simulink model "carmen_controller_forced"  (Simulink 8.2)
settings: Solver=FixedStepDiscrete  SolverMode=SingleTasking  StartTime=0.0  StopTime=inf  RelTol=1e-3
PreLoadFcn:
  | waijung.modelPreload; % Required for working with Waijung Blockset. Do not remove.
undefined symbols (not defined in the file or in its folder): ARM, Link, LQFP100, MDK, ST, STM32F407VG, STM32F4DISCOVERY
libraries: simulink x4, BC_USB x2, stm32f4_adc_lib x1, stm32f4_io_lib x1, stm32f4_device_config_lib x1
CloseFcn:
  | waijung.modelClose; % Required for working with Waijung Blockset. Do not remove.
settings Model: Creator=Sr Antonio  LastModifiedBy=Cristina
settings OptimizationCC: OptimizeModelRefInitCode=on  LifeSpan=1
settings DebuggingCC: FcnCallInpInsideContextMsg=EnableAllAsWarning
settings HardwareCC: ProdEndianess=LittleEndian  ProdHWDeviceType=ARM Compatible->Cortex - M4  TargetEndianess=LittleEndian  TargetHWDeviceType=ARM Compatible->Cortex - M4
settings RTWCC: SystemTargetFile=stm32f4.tlc  GenerateMakefile=off  TemplateMakefile=ert_default_tmf  Description=STM32F4 Target  ProcessScript=stm32f4_make_rtw_hook
settings CodeAppCC: IgnoreCustomStorageClasses=off  CustomSymbolStrType=$N$R$M  InternalIdentifier=Classic
settings STFCustomTargetCC: CodeReplacementLibrary=ANSI_C  ModelReferenceCompliant=off  CombineOutputUpdateFcns=on  ERTCustomFileBanners=on  SupportContinuousTime=off  SupportNonInlinedSFcns=off  MATLABClassNameForMDSCustomization=Simulink.SoftwareTarget.ERTCustomization  GRTInterface=off  SystemTargetFile=stm32f4.tlc
settings ERTTargetCC: CodeReplacementLibrary=ANSI_C  MultiwordLength=2048  ModelReferenceCompliant=off  ParMdlRefBuildCompliant=off  CompOptLevelCompliant=off  ConcurrentExecutionCompliant=off  ERTFirstTimeCompliant=off  ModelStepFunctionPrototypeControlCompliant=off  CPPClassGenCompliant=off  ExtModeMexFile=noextcomm  InlinedParameterPlacement=NonHierarchical  ERTSrcFileBannerTemplate=stm32f4_code_template.cgt  ERTHdrFileBannerTemplate=stm32f4_code_template.cgt  ERTDataSrcFileTemplate=stm32f4_code_template.cgt  ERTDataHdrFileTemplate=stm32f4_code_template.cgt  ERTCustomFileTemplate=stm32f4_file_process.tlc  ConvertIfToSwitch=off  SuppressUnreachableDefaultCases=off

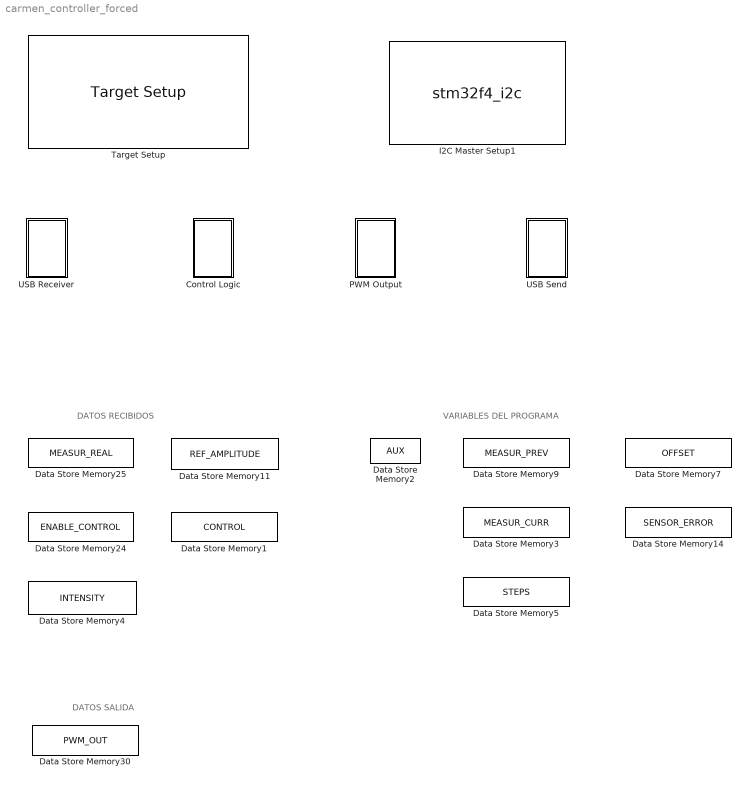
== system carmen_controller_forced ==
  note: VARIABLES DEL PROGRAMA
  note: DATOS RECIBIDOS
  note: DATOS SALIDA
  Control Logic : Subsystem  Priority=2
  Data Store Memory1 : DataStoreMemory  DataStoreName=CONTROL  ReadBeforeWriteMsg=warning  WriteAfterWriteMsg=warning  WriteAfterReadMsg=warning  OutDataTypeStr=single
  Data Store Memory11 : DataStoreMemory  DataStoreName=REF_AMPLITUDE  ReadBeforeWriteMsg=warning  WriteAfterWriteMsg=warning  WriteAfterReadMsg=warning  InitialValue=single(0)  OutDataTypeStr=single
  Data Store Memory14 : DataStoreMemory  DataStoreName=SENSOR_ERROR  ReadBeforeWriteMsg=warning  WriteAfterWriteMsg=warning  WriteAfterReadMsg=warning  OutDataTypeStr=uint8
  Data Store Memory2 : DataStoreMemory  DataStoreName=AUX  ReadBeforeWriteMsg=warning  WriteAfterWriteMsg=warning  WriteAfterReadMsg=warning  OutDataTypeStr=uint8
  Data Store Memory24 : DataStoreMemory  DataStoreName=ENABLE_CONTROL  ReadBeforeWriteMsg=warning  WriteAfterWriteMsg=warning  WriteAfterReadMsg=warning  OutDataTypeStr=uint8
  Data Store Memory25 : DataStoreMemory  DataStoreName=MEASUR_REAL  ReadBeforeWriteMsg=warning  WriteAfterWriteMsg=warning  WriteAfterReadMsg=warning  OutDataTypeStr=int32
  Data Store Memory3 : DataStoreMemory  DataStoreName=MEASUR_CURR  ReadBeforeWriteMsg=warning  WriteAfterWriteMsg=warning  WriteAfterReadMsg=warning  OutMin=0  OutMax=4096  OutDataTypeStr=uint16
  Data Store Memory30 : DataStoreMemory  DataStoreName=PWM_OUT  ReadBeforeWriteMsg=warning  WriteAfterWriteMsg=warning  WriteAfterReadMsg=warning  OutDataTypeStr=single
  Data Store Memory4 : DataStoreMemory  DataStoreName=INTENSITY  ReadBeforeWriteMsg=warning  WriteAfterWriteMsg=warning  WriteAfterReadMsg=warning  OutDataTypeStr=single
  Data Store Memory5 : DataStoreMemory  DataStoreName=STEPS  ReadBeforeWriteMsg=warning  WriteAfterWriteMsg=warning  WriteAfterReadMsg=warning  OutDataTypeStr=int8
  Data Store Memory7 : DataStoreMemory  DataStoreName=OFFSET  ReadBeforeWriteMsg=warning  WriteAfterWriteMsg=warning  WriteAfterReadMsg=warning  InitialValue=150  OutDataTypeStr=uint16
  Data Store Memory9 : DataStoreMemory  DataStoreName=MEASUR_PREV  ReadBeforeWriteMsg=warning  WriteAfterWriteMsg=warning  WriteAfterReadMsg=warning  OutMin=0  OutMax=4096  OutDataTypeStr=uint16
  I2C Master Setup1 : S-Function  Priority=2  FunctionName=stm32f4_i2c  Parameters=configuration,module,transfer,clkspeed,timeout,sdapin,sclpin,writecount,readcount,inputtypearray,outputtypearray,confstr,sampletime,sampletimestr,blockid  EnableBusSupport=off  mask(stm32f4_i2c){configuration=Setup, module=1, lastmodule=1, transfer=Blocking, dutycycle=TLow/THigh = 2, clkspeed=600, timeout=1, writecount=0, readcount=0, sdapin=B9, sclpin=B8, waitwritetime=0, inputtypearray=[0], outputtypearray=[0], confstr=["B","9","B","8","1","1","6","0","I2C_DutyCycle_2","0","off"], sampletime=-1, sampletimestr=0.002, blockid=I2CMasterSetup1}
      mask prompts: module "I2C Module"; lastmodule "Last module"; transfer "Transfer mode"; dutycycle "Duty cycle in fast mode"; clkspeed "Clock speed (kHz)"; timeout "Timeout (ms)"; writecount "Bytes write count"; readcount "Bytes read count"; sdapin "SDA pin"; sclpin "SCL pin"; waitwritetime "Wait write time (ms), default is 0"; inputtypearray "Input type array"; outputtypearray "Output type array"; confstr "Configuration string"; sampletime "Sample time (sec)"; sampletimestr "Compiled sample time (sec) in string"
      mask init:
      | stm32f4_i2c_callback('init');
      mask Help: web(fullfile(waijungdocroot,'stm32f4_i2c_setup.htm'), '-browser')
      mask TypeOptions configuration: Setup | Transaction
      mask Callback configuration: stm32f4_i2c_callback('configuration');
      mask TypeOptions module: 1 | 2 | 3
      mask Callback module: stm32f4_i2c_callback('module');
      mask TypeOptions transfer: Blocking | Non-blocking
      mask TypeOptions dutycycle: TLow/THigh = 16/9 | TLow/THigh = 2
      mask Callback dutycycle: stm32f4_i2c_callback('dutycycle');
      mask Callback writecount: stm32f4_i2c_callback('writecount');
      mask Callback readcount: stm32f4_i2c_callback('readcount');
      mask TypeOptions sdapin: - | B7 | B9
      mask Callback sdapin: stm32f4_i2c_callback('sdapin');
      mask TypeOptions sclpin: - | B6 | B8
      mask Callback sclpin: stm32f4_i2c_callback('sclpin');
      mask Callback confstr: stm32f4_i2c_callback('confstr');
      mask Callback sampletime: stm32f4_i2c_callback('sampletime');
      mask Callback sampletimestr: stm32f4_i2c_callback('sampletimestr');
      mask Callback blockid: stm32f4_i2c_callback('blockid');
      mask Display: text(0.5, 0.5, 'Module: I2C1\nClock: 600kHz\nSDA/SCL Pin: B9/B8','ver','middle','hor','center');
  PWM Output : Subsystem  Priority=3
  Target Setup : stm32f4_device_config_lib/Target Setup  Priority=1  compiler=MDK-ARM  previous_compiler=MDK-ARM  mcu=STM32F407VG (LQFP100); STM32F4DISCOVERY  mcustr=STM32F407VG  clockconfig=STM32F4DISCOVERY Default (HSEOSC-8MHz/HCLK-168MHz)  system_stm32f4xx_c_path=C:\BC_3\targets\stm32f4_target\stm32f4\utils\STM32F4xx_AN3988_V1.0.1\stm32f4_default\hseosc8mhz  showmemoryconfiguration=on  stacksize=0x1600  heapsize=0x1600  enableautocompiledownload=on  fullchiperase=off  programmerinterface=ST-Link  editctrlstr=on  compilercontrolstr=-c --cpu Cortex-M4.fp -g -O3 --apcs=interwork --split_sections $(INCLUDES)  assemblercontrolstr="--cpu Cortex-M4.fp -g --apcs=interwork  --xref $(INCLUDES)"  linkercontrolstr="--cpu Cortex-M4.fp --strict --scatter \"$(MODELNAME).sct\" --summary_stderr --info summarysizes --map --xref --callgraph --symbols --info sizes --info totals --info unused --info veneers  --list \".\\$(MODELNAME).map\" -o $(MODELNAME).axf"  runafterdownload=on  execprofile=None  profileruart=3  profilerbaud=500000  profilertxpin=D8  profilerinitstr=0.002,168000000,336000,500000,0  manualsetsampletime=on  sampletime=0.002  blockid=TargetSetup  systickreloadvalue=336000  hseval=8000000  lastprofileruart=3  hclk=168000000  flashorigin=0x08000000  flashlength=0x00100000  ramorigin=0x20000000  ramlength=0x00020000  useextram=off
  USB Receiver : Subsystem  Priority=4
  USB Send : Subsystem  Priority=5

== system carmen_controller_forced/Control Logic ==
  Read Sensor : Subsystem  Priority=2

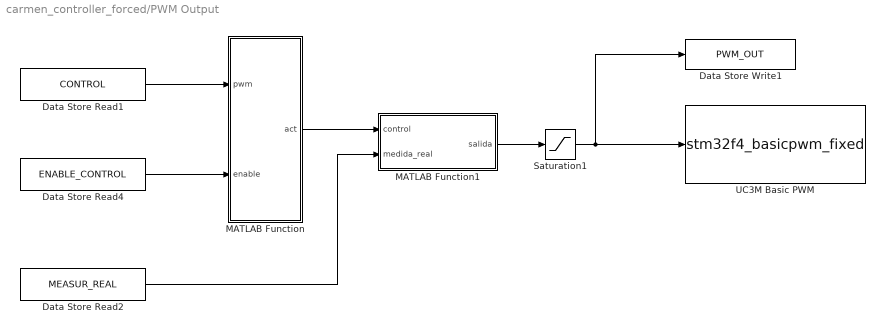
== system carmen_controller_forced/PWM Output ==
  Data Store Read1 : DataStoreRead  DataStoreName=CONTROL
  Data Store Read2 : DataStoreRead  DataStoreName=MEASUR_REAL
  Data Store Read4 : DataStoreRead  DataStoreName=ENABLE_CONTROL
  Data Store Write1 : DataStoreWrite  DataStoreName=PWM_OUT
  MATLAB Function : MATLAB Function  TreatAsAtomicUnit=on
  MATLAB Function1 : MATLAB Function  TreatAsAtomicUnit=on
  Saturation1 : Saturate  UpperLimit=100  LowerLimit=0  OutDataTypeStr=single
  UC3M Basic PWM : S-Function  Priority=6  FunctionName=stm32f4_basicpwm_fixed  Parameters=timer,pwmperiod,uc3m_pwmperiod,ch1pin,ch2pin,ch3pin,ch4pin,sampletime,sampletimestr,blockid,apb,portstr,pinstr,pinmat,timarr,timprescale,chmat,polaritystr  EnableBusSupport=off  mask(stm32f4_basicpwm_fixed){timer=2, pwmperiod=0.02, uc3m_pwmperiod=0.001, polarity=Active High, polaritystr=TIM_OCPolarity_High, ch1pin=Not available - Do not use, ch2pin=B3, ch3pin=Not available - Do not use, ch4pin=Not available - Do not use, sampletime=0.002, sampletimestr=0, blockid=PWMOutputUC3MBasicPWM, portpinstr=,B3,,, enablecustomportlabel=off, cinputportlabel=In1, In2, In3, In4, coutputportlabel=0, callbackgensrccode=off, apb=1, portstr=["B"], pinstr=["GPIO_Pin_3"], pinmat=[1 3], timarr=59999, timprescale=55, chmat=[2]}
      mask prompts: pwmperiod "PWM Period (seconds)"; uc3m_pwmperiod "PWM Signal Period (seconds)"; ch1pin "Channel 1"; ch2pin "Channel 2"; ch3pin "Channel 3"; ch4pin "Channel 4"; sampletime "Sample time (sec)"; sampletimestr "Compiled sample time (sec) in string"; portpinstr "Port pin string"; enablecustomportlabel "Enable custom port labels"; cinputportlabel "Custom input port labels (Ex. In1, In2, In3)"; coutputportlabel "Custom output port labels (Ex. Out1, Out2, Out3)"; callbackgensrccode "Gen source code from callback"; portstr "Port string"; pinstr "Pin string"; pinmat "Pin matrix"; timarr "Timer ARR"; timprescale "Timer PRESCALE"; chmat "Channel order"
      mask help:
      | This block implements basic Edge-aligned Pulse Width Modulation (PWM) generation.
      | All timers are 16-bit. The PWM period is fixed (per timer).
      |
      | This block was fixed by Sr Antonio
      mask init:
      | stm32f4_basicpwm_callback_fixed('init');
      mask Help: web(fullfile(waijungdocroot,'stm32f4_basicpwm.htm'),'-browser')
      mask TypeOptions timer: 1 | 2 | 3 | 4 | 5 | 8 | 9 | 10 | 11 | 12 | 13 | 14
      mask Callback timer: stm32f4_basicpwm_callback_fixed('timer');
      mask Callback pwmperiod: stm32f4_basicpwm_callback_fixed('pwmperiod');
      mask Callback uc3m_pwmperiod: stm32f4_basicpwm_callback_fixed('uc3m_pwmperiod');
      mask TypeOptions polarity: Active High | Active Low
      mask Callback polarity: stm32f4_basicpwm_callback_fixed('polarity');
      mask TypeOptions ch1pin: Not available - Do not use | A0 | A5
      mask Callback ch1pin: stm32f4_basicpwm_callback_fixed('ch1pin');
      mask TypeOptions ch2pin: Not available - Do not use | A1 | B3
      mask Callback ch2pin: stm32f4_basicpwm_callback_fixed('ch2pin');
      mask TypeOptions ch3pin: Not available - Do not use | A2 | B10
      mask Callback ch3pin: stm32f4_basicpwm_callback_fixed('ch3pin');
      mask TypeOptions ch4pin: Not available - Do not use | A3 | B11
      mask Callback ch4pin: stm32f4_basicpwm_callback_fixed('ch4pin');
      mask Callback sampletime: stm32f4_basicpwm_callback_fixed('sampletime');
      mask Callback sampletimestr: stm32f4_basicpwm_callback_fixed('sampletimestr');
      mask Callback blockid: stm32f4_basicpwm_callback_fixed('blockid');
      mask Callback enablecustomportlabel: stm32f4_basicpwm_callback_fixed('enablecustomportlabel')
      mask Display: text(0.95, 0.5, 'UC3M FIXED\nTimer: 2\nPolarity: Active High\nPeriod (sec): 0.001\nTs (sec): 0.002','ver','middle','hor','right');port_label('input', 1,'CH2 (B3)')
  wires:
  Data Store Read1/1 -> MATLAB Function/1(pwm)
  Data Store Read4/1 -> MATLAB Function/2(enable)
  MATLAB Function/1(act) -> MATLAB Function1/1(control)
  Saturation1/1 -> UC3M Basic PWM/1, Data Store Write1/1
  Data Store Read2/1 -> MATLAB Function1/2(medida_real)
  MATLAB Function1/1(salida) -> Saturation1/1

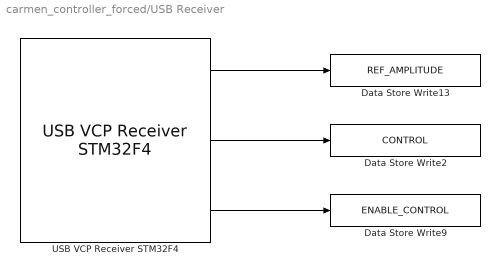
== system carmen_controller_forced/USB Receiver ==
  Data Store Write13 : DataStoreWrite  DataStoreName=REF_AMPLITUDE
  Data Store Write2 : DataStoreWrite  DataStoreName=CONTROL
  Data Store Write9 : DataStoreWrite  DataStoreName=ENABLE_CONTROL
  USB VCP Receiver STM32F4 : BC_USB/USB VCP Receiver STM32F4  speed="USB 1.1   12Mbit/s"  data_size=2048 Bytes  header_data='0E 0E'  binary_data='single single uint8'  terminator_data='0A 0A'  sampletime=0.01
  wires:
  USB VCP Receiver STM32F4/1 -> Data Store Write13/1
  USB VCP Receiver STM32F4/2 -> Data Store Write2/1
  USB VCP Receiver STM32F4/3 -> Data Store Write9/1

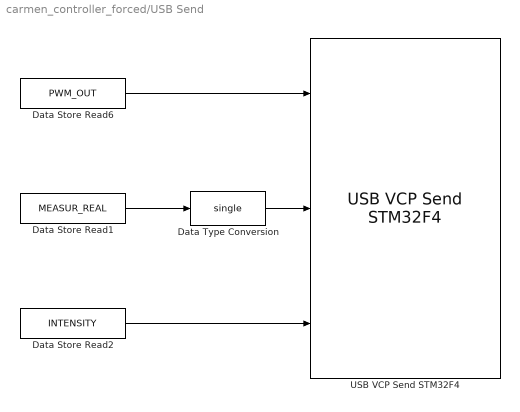
== system carmen_controller_forced/USB Send ==
  Data Store Read1 : DataStoreRead  DataStoreName=MEASUR_REAL  SampleTime=0.002
  Data Store Read2 : DataStoreRead  DataStoreName=INTENSITY  SampleTime=0.01
  Data Store Read6 : DataStoreRead  DataStoreName=PWM_OUT  SampleTime=0.002
  Data Type Conversion : DataTypeConversion  OutDataTypeStr=single
  USB VCP Send STM32F4 : BC_USB/USB VCP Send STM32F4  speed="USB 1.1   12Mbit/s"  data_size=2048 Bytes  header_data='0E 0E'  binary_data='single single single'  terminator_data='0A 0A'  sampletime=0.01
  wires:
  Data Store Read1/1 -> Data Type Conversion/1
  Data Store Read6/1 -> USB VCP Send STM32F4/1
  Data Type Conversion/1 -> USB VCP Send STM32F4/2
  Data Store Read2/1 -> USB VCP Send STM32F4/3

== system carmen_controller_forced/Control Logic/Read Sensor ==
  note: LECTURA DEL SENSOR DE INTENSIDAD
  note: CÁLCULO DE LA POSICIÓN REAL DEL ACTUADOR
  note: LECTURA DEL SENSOR DE POSICIÓN
  Calculate the SMA real position : Subsystem  Priority=3
  Intensity Readout : Subsystem  Priority=2
  Sensor Readout : Subsystem  Priority=2

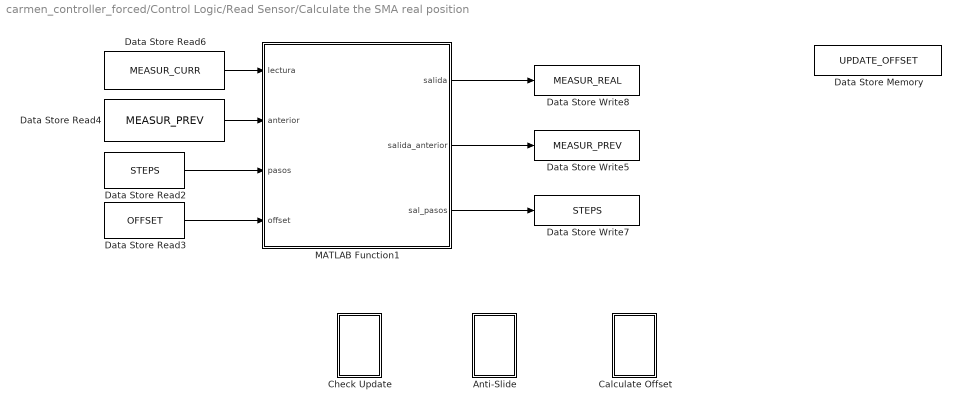
== system carmen_controller_forced/Control Logic/Read Sensor/Calculate the SMA real position ==
  Anti-Slide : Subsystem  Priority=51
  Calculate Offset : Subsystem  Priority=52
  Check Update : Subsystem  Priority=50
  Data Store Memory : DataStoreMemory  DataStoreName=UPDATE_OFFSET  ReadBeforeWriteMsg=warning  WriteAfterWriteMsg=warning  WriteAfterReadMsg=warning  OutDataTypeStr=uint8
  Data Store Read2 : DataStoreRead  DataStoreName=STEPS  SampleTime=0.002
  Data Store Read3 : DataStoreRead  DataStoreName=OFFSET  SampleTime=0.002
  Data Store Read4 : DataStoreRead  DataStoreName=MEASUR_PREV  SampleTime=0.002
  Data Store Read6 : DataStoreRead  DataStoreName=MEASUR_CURR  SampleTime=0.002
  Data Store Write5 : DataStoreWrite  DataStoreName=MEASUR_PREV  SampleTime=0.002
  Data Store Write7 : DataStoreWrite  DataStoreName=STEPS  SampleTime=0.002
  Data Store Write8 : DataStoreWrite  DataStoreName=MEASUR_REAL  SampleTime=0.002
  MATLAB Function1 : MATLAB Function  TreatAsAtomicUnit=on
  wires:
  Data Store Read2/1 -> MATLAB Function1/3(pasos)
  Data Store Read4/1 -> MATLAB Function1/2(anterior)
  MATLAB Function1/3(sal_pasos) -> Data Store Write7/1
  Data Store Read6/1 -> MATLAB Function1/1(lectura)
  MATLAB Function1/1(salida) -> Data Store Write8/1
  MATLAB Function1/2(salida_anterior) -> Data Store Write5/1
  Data Store Read3/1 -> MATLAB Function1/4(offset)

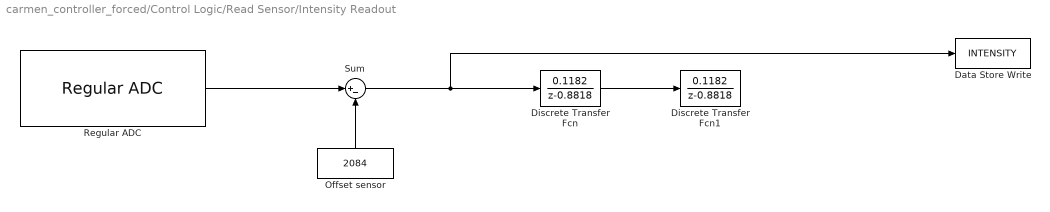
== system carmen_controller_forced/Control Logic/Read Sensor/Intensity Readout ==
  Data Store Write : DataStoreWrite  DataStoreName=INTENSITY
  Discrete Transfer Fcn : DiscreteTransferFcn  Numerator=[0.1182]  Denominator=[1 -0.8818]
  Discrete Transfer Fcn1 : DiscreteTransferFcn  Numerator=[0.1182]  Denominator=[1 -0.8818]
  Offset sensor : Constant  Value=2084  OutDataTypeStr=single
  Regular ADC : stm32f4_adc_lib/Regular ADC  adcmodule=1  outputdatatype=Single  prescaler=2  prescalerstr=ADC_Prescaler_Div2  chsamplingtime=Auto  chsamplingtimestr=ADC_SampleTime_480Cycles  read_an0=off  read_an1=off  read_an2=on  read_an3=off  read_an4=off  read_an5=off  read_an6=off  read_an7=off  read_an8=off  read_an9=off  read_an10=off  read_an11=off  read_an12=off  read_an13=off  read_an14=off  read_an15=off  read_an16=off  read_an17=off  read_an18=off  pinstr=GPIO_Pin_2  usedpinarray="[0  0  1  0  0  0  0  0  0  0  0  0  0  0  0  0  0  0  0]"  usedportidarray=[0]  usedpinidarray=[2]  usedpinidcount=1  sampletime=0.002  blockid=ControlLogicReadSensorIntensityReadoutRegularADC  enablecustomportlabel=off  cinputportlabel=0  coutputportlabel=Out1, Out2
  Sum : Sum  Inputs=|+-
  wires:
  Discrete Transfer Fcn/1 -> Discrete Transfer Fcn1/1
  Regular ADC/1 -> Sum/1
  Sum/1 -> Data Store Write/1, Discrete Transfer Fcn/1
  Offset sensor/1 -> Sum/2

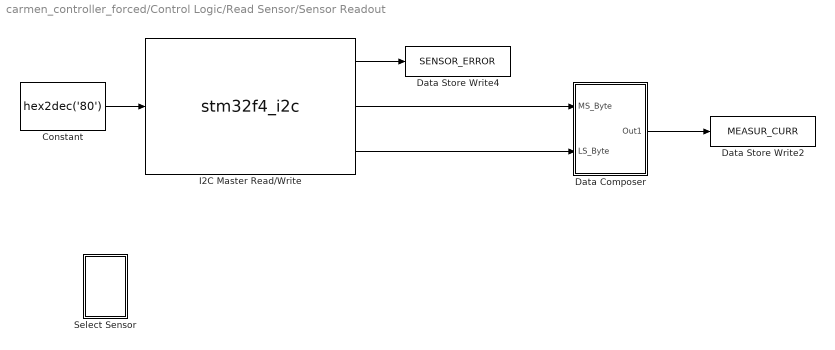
== system carmen_controller_forced/Control Logic/Read Sensor/Sensor Readout ==
  Constant : Constant  Value=hex2dec('80')  OutDataTypeStr=uint8  SampleTime=-1
  Data Composer : Subsystem  Priority=3
  Data Store Write2 : DataStoreWrite  Priority=3  DataStoreName=MEASUR_CURR  SampleTime=0.002
  Data Store Write4 : DataStoreWrite  Priority=4  DataStoreName=SENSOR_ERROR  SampleTime=0.002
  I2C Master Read/Write : S-Function  FunctionName=stm32f4_i2c  Parameters=configuration,module,transfer,clkspeed,timeout,sdapin,sclpin,writecount,readcount,inputtypearray,outputtypearray,confstr,sampletime,sampletimestr,blockid  EnableBusSupport=off  mask(stm32f4_i2c){configuration=Transaction, module=1, lastmodule=3, transfer=Blocking, dutycycle=TLow/THigh = 2, clkspeed=400, timeout=25, writecount=0, readcount=2, sdapin=C9, sclpin=A8, waitwritetime=0, inputtypearray=[1 3], outputtypearray=[3 3 3 3], confstr=["C","9","A","8","1","1","6","0","I2C_DutyCycle_2","0","off"], sampletime=-1, sampletimestr=0.002, blockid=ControlLogicReadSensorSensorReadoutI2CMasterReadWrite}
      mask prompts: module "I2C Module"; lastmodule "Last module"; transfer "Transfer mode"; dutycycle "Duty cycle in fast mode"; clkspeed "Clock speed (kHz)"; timeout "Timeout (ms)"; writecount "Bytes write count"; readcount "Bytes read count"; sdapin "SDA pin"; sclpin "SCL pin"; waitwritetime "Wait write time (ms), default is 0"; inputtypearray "Input type array"; outputtypearray "Output type array"; confstr "Configuration string"; sampletime "Sample time (sec)"; sampletimestr "Compiled sample time (sec) in string"
      mask help:
      | SlvAddr:
      |  - I2C device address, left justify (R/W bit append to bit 0).
      |  - For I2C Read transaction, the block will adjust bit 0 of device address to '1' automatically.
      | Status:
      |  - Output port represent the status of transaction.
      |  - Status = 0, Success.
      |    Status = 1, Error NAK.
      |    Status = 2, Error Timeout.
      mask init:
      | stm32f4_i2c_callback('init');
      mask Help: web(fullfile(waijungdocroot,'stm32f4_i2c_readwrite.htm'), '-browser')
      mask TypeOptions configuration: Setup | Transaction
      mask Callback configuration: stm32f4_i2c_callback('configuration');
      mask TypeOptions module: 1 | 2 | 3
      mask Callback module: stm32f4_i2c_callback('module');
      mask TypeOptions transfer: Blocking | Non-blocking
      mask TypeOptions dutycycle: TLow/THigh = 16/9 | TLow/THigh = 2
      mask Callback dutycycle: stm32f4_i2c_callback('dutycycle');
      mask Callback writecount: stm32f4_i2c_callback('writecount');
      mask Callback readcount: stm32f4_i2c_callback('readcount');
      mask TypeOptions sdapin: - | C9
      mask Callback sdapin: stm32f4_i2c_callback('sdapin');
      mask TypeOptions sclpin: - | A8
      mask Callback sclpin: stm32f4_i2c_callback('sclpin');
      mask Callback confstr: stm32f4_i2c_callback('confstr');
      mask Callback sampletime: stm32f4_i2c_callback('sampletime');
      mask Callback sampletimestr: stm32f4_i2c_callback('sampletimestr');
      mask Callback blockid: stm32f4_i2c_callback('blockid');
      mask Display: text(0.5, 0.5, 'Module: I2C1\nTransfer: Blocking\nWrite: 0 bytes\nRead: 2 bytes\nTs (sec): 0.002','ver','middle','hor','center');port_label('input', 1,'SlvAddr');port_label('output', 1,'Status');port_label('output', 2,'Rd0 (uint8)');port_label('output', 3,'Rd1 (uint8)');
  Select Sensor : Subsystem  Priority=1
  wires:
  Constant/1 -> I2C Master Read/Write/1
  I2C Master Read/Write/2 -> Data Composer/1(MS_Byte)
  I2C Master Read/Write/3 -> Data Composer/2(LS_Byte)
  I2C Master Read/Write/1 -> Data Store Write4/1
  Data Composer/1(Out1) -> Data Store Write2/1

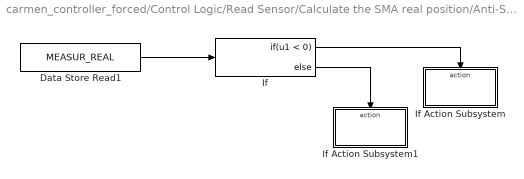
== system carmen_controller_forced/Control Logic/Read Sensor/Calculate the SMA real position/Anti-Slide ==
  Data Store Read1 : DataStoreRead  DataStoreName=MEASUR_REAL  SampleTime=0.002
  If : If  IfExpression=u1 < 0
  If Action Subsystem : Subsystem  TreatAsAtomicUnit=on
  If Action Subsystem1 : Subsystem  TreatAsAtomicUnit=on
  wires:
  Data Store Read1/1 -> If/1
  If/1 -> If Action Subsystem/Action
  If/2 -> If Action Subsystem1/Action

== system carmen_controller_forced/Control Logic/Read Sensor/Calculate the SMA real position/Calculate Offset ==
  Data Store Read1 : DataStoreRead  Priority=4  DataStoreName=AUX
  If : If  IfExpression=u1 == 0  ShowElse=off
  If Action Subsystem : Subsystem  TreatAsAtomicUnit=on
  wires:
  Data Store Read1/1 -> If/1
  If/1 -> If Action Subsystem/Action

== system carmen_controller_forced/Control Logic/Read Sensor/Calculate the SMA real position/Check Update ==
  Data Store Read5 : DataStoreRead  DataStoreName=UPDATE_OFFSET  SampleTime=0.002
  If Action Subsystem2 : Subsystem  TreatAsAtomicUnit=on
  If1 : If  IfExpression=u1 == 210  ShowElse=off
  wires:
  Data Store Read5/1 -> If1/1
  If1/1 -> If Action Subsystem2/Action

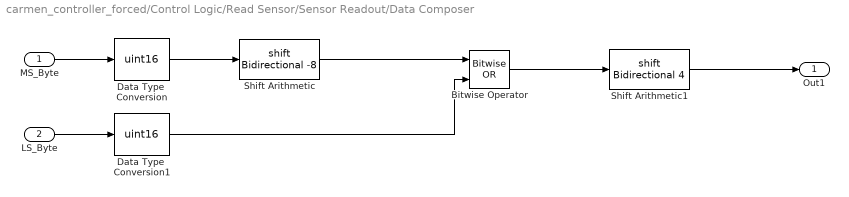
== system carmen_controller_forced/Control Logic/Read Sensor/Sensor Readout/Data Composer ==
  MS_Byte : Inport  OutDataTypeStr=uint8
  LS_Byte : Inport  Port=2  OutDataTypeStr=uint8
  Bitwise Operator : simulink/Logic and Bit Operations/Bitwise Operator  logicop=OR  UseBitMask=off  NumInputPorts=2  BitMask=bin2dec('11011001')  BitMaskRealWorld=Stored Integer
  Data Type  Conversion : DataTypeConversion  OutDataTypeStr=uint16  SaturateOnIntegerOverflow=on  RndMeth=Zero
  Data Type  Conversion1 : DataTypeConversion  OutDataTypeStr=uint16  SaturateOnIntegerOverflow=on  RndMeth=Zero
  Shift Arithmetic : ArithShift  BitShiftNumber=-8
  Shift Arithmetic1 : ArithShift  BitShiftNumber=4
  Out1 : Outport  OutDataTypeStr=uint16
  wires:
  Shift Arithmetic1/1 -> Out1/1
  Bitwise Operator/1 -> Shift Arithmetic1/1
  Data Type  Conversion1/1 -> Bitwise Operator/2
  Shift Arithmetic/1 -> Bitwise Operator/1
  Data Type  Conversion/1 -> Shift Arithmetic/1
  LS_Byte/1 -> Data Type  Conversion1/1
  MS_Byte/1 -> Data Type  Conversion/1

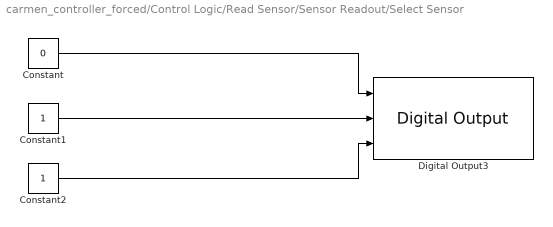
== system carmen_controller_forced/Control Logic/Read Sensor/Sensor Readout/Select Sensor ==
  Constant : Constant  Value=0  OutDataTypeStr=boolean  SampleTime=-1
  Constant1 : Constant  OutDataTypeStr=boolean  SampleTime=-1
  Constant2 : Constant  OutDataTypeStr=boolean  SampleTime=-1
  Digital Output3 : stm32f4_io_lib/Digital Output  use_bitband=on  port=A  speed=100  porttype=Push Pull  porttypestr=PP  use_pin0=off  use_pin1=off  use_pin2=off  use_pin3=off  use_pin4=on  use_pin5=on  use_pin6=on  use_pin7=off  use_pin8=off  use_pin9=off  use_pin10=off  use_pin11=off  use_pin12=off  use_pin13=off  use_pin14=off  use_pin15=off  pinstr=GPIO_Pin_4 | GPIO_Pin_5 | GPIO_Pin_6  usedpinarray="[0  0  0  0  1  1  1  0  0  0  0  0  0  0  0  0]"  bitbandingstr=|  sampletime=-1  sampletimestr=0  blockid=ControlLogicReadSensorSensorReadoutSelectSensorDigitalOutput3  enablecustomportlabel=off  globalinit=off  cinputportlabel=In1, In2  coutputportlabel=0
      | #define ControlLogicReadSensorSensorReadoutSelectSensorDigitalOutput3_A4 Peripheral_BB(GPIOA->ODR, 4)  /* Output pin */
      | #define ControlLogicReadSensorSensorReadoutSelectSensorDigitalOutput3_A5 Peripheral_BB(GPIOA->ODR, 5)  /* Output pin */
      | #define ControlLogicReadSensorSensorReadoutSelectSensorDigitalOutput3_A6 Peripheral_BB(GPIOA->ODR, 6)  /* Output pin */
  wires:
  Constant/1 -> Digital Output3/1
  Constant1/1 -> Digital Output3/2
  Constant2/1 -> Digital Output3/3

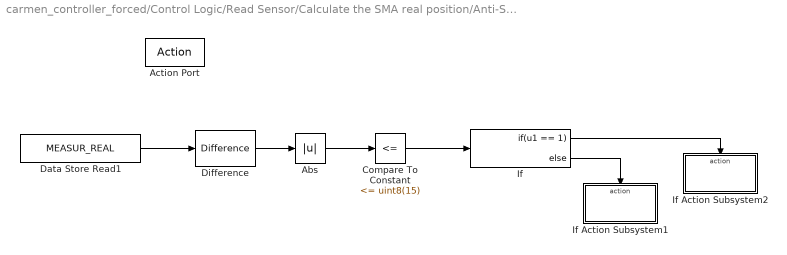
== system carmen_controller_forced/Control Logic/Read Sensor/Calculate the SMA real position/Anti-Slide/If Action Subsystem ==
  Action Port : ActionPort  ActionType=then
  Abs : Abs
  Compare To Constant : simulink/Logic and Bit Operations/Compare To Constant  relop=<=  const=uint8(15)  OutDataTypeStr=uint8
  Data Store Read1 : DataStoreRead  DataStoreName=MEASUR_REAL  SampleTime=0.002
  Difference : simulink/Discrete/Difference  ICPrevInput=0.0  InputProcessing=Inherited  OutMin=[]  OutMax=[]  OutDataType=fixdt(1, 16)  OutScaling=2^-10  DoSatur=off
  If : If  IfExpression=u1 == 1
  If Action Subsystem1 : Subsystem  TreatAsAtomicUnit=on
  If Action Subsystem2 : Subsystem  TreatAsAtomicUnit=on
  wires:
  Data Store Read1/1 -> Difference/1
  Difference/1 -> Abs/1
  Abs/1 -> Compare To Constant/1
  Compare To Constant/1 -> If/1
  If/2 -> If Action Subsystem1/Action
  If/1 -> If Action Subsystem2/Action

== system carmen_controller_forced/Control Logic/Read Sensor/Calculate the SMA real position/Anti-Slide/If Action Subsystem1 ==
  Action Port : ActionPort  ActionType=else
  Constant : Constant  Value=0  OutDataTypeStr=uint8  SampleTime=-1
  Data Store Write : DataStoreWrite  DataStoreName=UPDATE_OFFSET
  wires:
  Constant/1 -> Data Store Write/1

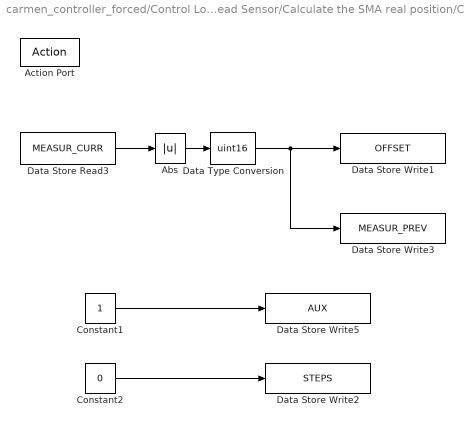
== system carmen_controller_forced/Control Logic/Read Sensor/Calculate the SMA real position/Calculate Offset/If Action Subsystem ==
  Action Port : ActionPort  ActionType=then
  Abs : Abs
  Constant1 : Constant  OutDataTypeStr=uint8  SampleTime=-1
  Constant2 : Constant  Value=0  OutDataTypeStr=int8  SampleTime=-1
  Data Store Read3 : DataStoreRead  Priority=4  DataStoreName=MEASUR_CURR
  Data Store Write1 : DataStoreWrite  Priority=4  DataStoreName=OFFSET
  Data Store Write2 : DataStoreWrite  Priority=4  DataStoreName=STEPS
  Data Store Write3 : DataStoreWrite  Priority=4  DataStoreName=MEASUR_PREV
  Data Store Write5 : DataStoreWrite  Priority=4  DataStoreName=AUX
  Data Type Conversion : DataTypeConversion  OutDataTypeStr=uint16
  wires:
  Data Store Read3/1 -> Abs/1
  Constant1/1 -> Data Store Write5/1
  Abs/1 -> Data Type Conversion/1
  Data Type Conversion/1 -> Data Store Write3/1, Data Store Write1/1
  Constant2/1 -> Data Store Write2/1

== system carmen_controller_forced/Control Logic/Read Sensor/Calculate the SMA real position/Check Update/If Action Subsystem2 ==
  Action Port : ActionPort  ActionType=then
  Constant : Constant  Value=0  OutDataTypeStr=uint8  SampleTime=-1
  Data Store Write : DataStoreWrite  DataStoreName=UPDATE_OFFSET
  Data Store Write1 : DataStoreWrite  DataStoreName=AUX
  wires:
  Constant/1 -> Data Store Write/1, Data Store Write1/1

== system carmen_controller_forced/Control Logic/Read Sensor/Calculate the SMA real position/Anti-Slide/If Action Subsystem/If Action Subsystem1 ==
  Action Port : ActionPort  ActionType=else
  Constant : Constant  Value=0  OutDataTypeStr=uint8  SampleTime=-1
  Data Store Write : DataStoreWrite  DataStoreName=UPDATE_OFFSET
  wires:
  Constant/1 -> Data Store Write/1

== system carmen_controller_forced/Control Logic/Read Sensor/Calculate the SMA real position/Anti-Slide/If Action Subsystem/If Action Subsystem2 ==
  Action Port : ActionPort  ActionType=then
  Data Store Read : DataStoreRead  DataStoreName=UPDATE_OFFSET
  Data Store Write : DataStoreWrite  DataStoreName=UPDATE_OFFSET
  Increment Stored Integer : simulink/Additional Math & Discrete/Additional Math: Increment - Decrement/Increment Stored Integer
  wires:
  Increment Stored Integer/1 -> Data Store Write/1
  Data Store Read/1 -> Increment Stored Integer/1

== matlab function Control Logic/Read Sensor/Calculate the SMA real position/MATLAB Function1 ==
  data: lectura input uint16; anterior input uint16; salida output int32; salida_anterior output uint16; pasos input int8; offset input uint16; sal_pasos output int8
function [salida,salida_anterior,sal_pasos] = fcn(lectura,anterior,pasos,offset)
%#codegen

salida_anterior=uint16(lectura);

if(lectura>3500)
    if(anterior<1000)
      pasos = int8(pasos + 1);     
    end
end

if(lectura<1000)
    if(anterior>3500)
      pasos = int8(pasos - 1);
      %if(pasos>250)
      %   pasos=uint8(0); 
      %end
    end
end
sal_pasos=int8(pasos);    

if(pasos==0)
   salida=int32(int32(offset)-int32(lectura)); 
else
   salida=int32(int32(offset)+(4096*int32(pasos))-int32(lectura)); 
end

== matlab function PWM Output/MATLAB Function ==
  data: pwm input double; act output double; enable input double
function act  = fcn(pwm,enable)
%#codegen

if enable==uint8(0)
    act=single(0);
else
    act=pwm;
end

== matlab function PWM Output/MATLAB Function1 ==
  data: control input double; medida_real input double; salida output double
function salida = fcn(control, medida_real)
%#codegen

if medida_real>single(75000)
    salida=single(0); 
else
    salida = control;
end
